simulink model "v3_sim_lqi_sigma_x1_time_variant"  (R2023b)
settings: Solver=VariableStepAuto  StartTime=0.0  StopTime=180  RelTol=1e-10
values from neighbouring files (symbols this model uses):
  K_sigma = [K_sigma, K.']    [WP5.m]
  sigma = [0.01:0.02:2]    [WP5.m]
undefined symbols (not defined in the file or in its folder): reference_selector
libraries: simulink x3
settings Model: Creator=kiraa  LastModifiedBy=kiraa

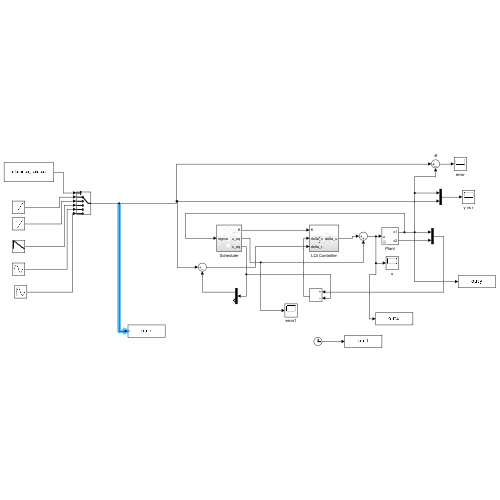
[thumbnail: Simulink's stored preview of the top-level diagram]
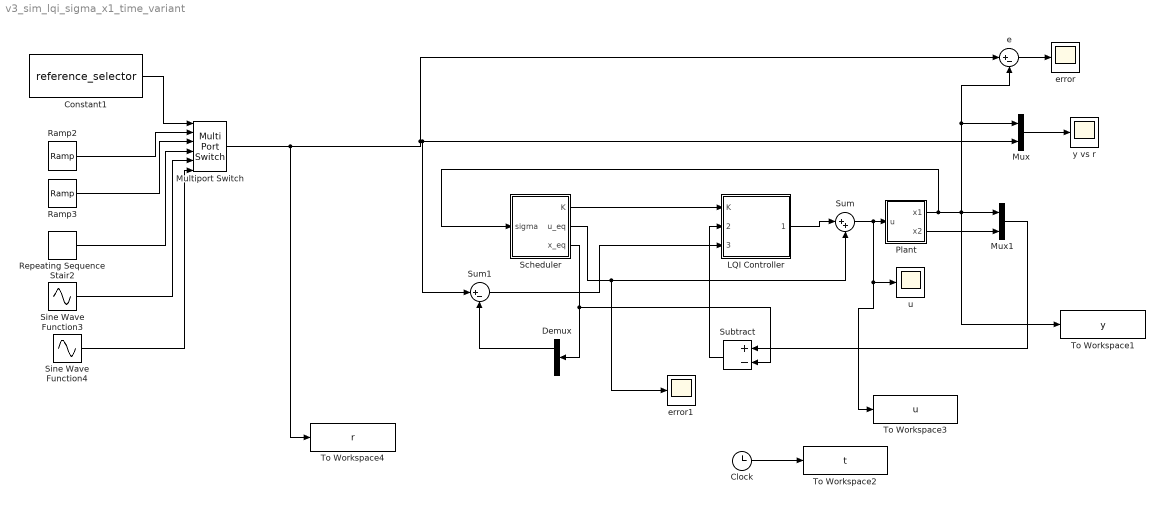
== system v3_sim_lqi_sigma_x1_time_variant ==
  Clock : Clock
  Constant1 : Constant  Value=reference_selector
  Demux : Demux  Outputs=2
  LQI Controller : Subsystem
  Multiport Switch : MultiPortSwitch  Inputs=5  SaturateOnIntegerOverflow=off  InputSameDT=off
  Mux : Mux  Inputs=2
  Mux1 : Mux  Inputs=2
  Plant : Subsystem  mask{x1_0=0.1, x2_0=0}
      mask prompts: x1_0 "x1(0) [g/l]"; x2_0 "x2(0) [min^-1]"
  Ramp2 : simulink/Sources/Ramp  slope=-0.0005  start=0  InitialOutput=0.1
  Ramp3 : simulink/Sources/Ramp  slope=0.005  start=0  InitialOutput=0.1
  Repeating Sequence Stair2 : simulink/Sources/Repeating Sequence Stair  OutValues=[ 0.085 0.08 0.075 0.07 0.065 0.06 0.055 0.05 0.045 0.04 0.035 0.03].'  tsamp=20  OutMin=[]  OutMax=[]  OutDataTypeStr=double  OutputDataTypeScalingMode=double  OutDataType=fixdt(0,8)  ConRadixGroup=Best Precision: Vector-wise  OutScaling=2^-12
  Scheduler : Subsystem
  Sine Wave Function3 : Sin  Amplitude=0.03  Bias=0.05  Frequency=0.05  SampleTime=0
  Sine Wave Function4 : Sin  Amplitude=0.02  Bias=0.05  Frequency=0.1  SampleTime=0
  Subtract : Sum  Inputs=+-
  Sum : Sum  Inputs=|++
  Sum1 : Sum  Inputs=|+-
  To Workspace1 : ToWorkspace  VariableName=y  SampleTime=-1
  To Workspace2 : ToWorkspace  VariableName=t  SampleTime=-1
  To Workspace3 : ToWorkspace  VariableName=u  SampleTime=-1
  To Workspace4 : ToWorkspace  VariableName=r  SampleTime=-1
  e : Sum  Inputs=|+-
  error : Scope
  error1 : Scope
  u : Scope
  y vs r : Scope
  wires:
  Mux/1 -> y vs r/1
  Plant/1(x1) -> Scheduler/1(sigma), To Workspace1/1, Mux/1, e/2, Mux1/1
  LQI Controller/1(delta_u) -> Sum/1
  e/1 -> error/1
  Sum/1 -> To Workspace3/1, u/1, Plant/1(u)
  Subtract/1 -> LQI Controller/2(delta_x)
  Plant/2(x2) -> Mux1/2
  Mux1/1 -> Subtract/1
  Scheduler/2(u_eq) -> error1/1, Sum/2
  Scheduler/3(x_eq) -> Subtract/2, Demux/1
  Scheduler/1(K) -> LQI Controller/1(K)
  Demux/1 -> Sum1/2
  Sum1/1 -> LQI Controller/3(delta_r)
  Clock/1 -> To Workspace2/1
  Sine Wave Function4/1 -> Multiport Switch/6
  Repeating Sequence Stair2/1 -> Multiport Switch/4
  Constant1/1 -> Multiport Switch/1
  Ramp3/1 -> Multiport Switch/3
  Ramp2/1 -> Multiport Switch/2
  Sine Wave Function3/1 -> Multiport Switch/5
  Multiport Switch/1 -> To Workspace4/1, e/1, Mux/2, Sum1/1

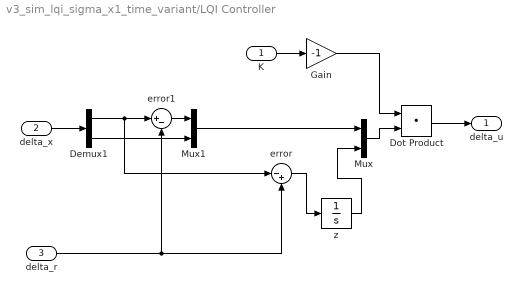
== system v3_sim_lqi_sigma_x1_time_variant/LQI Controller ==
  K : Inport
  delta_x : Inport  Port=2
  delta_r : Inport  Port=3
  Demux1 : Demux  Outputs=2
  Dot Product : DotProduct  OutDataTypeStr=Inherit: Inherit via internal rule
  Gain : Gain  Gain=-1
  Mux : Mux  Inputs=2
  Mux1 : Mux  Inputs=2
  error : Sum  Inputs=|-+
  error1 : Sum  Inputs=|+-
  z : Integrator  InitialCondition=0.1
  delta_u : Outport
  wires:
  Gain/1 -> Dot Product/1
  delta_r/1 -> error1/2, error/2
  Demux1/1 -> error1/1, error/1
  Mux1/1 -> Mux/1
  error/1 -> z/1
  z/1 -> Mux/2
  K/1 -> Gain/1
  Mux/1 -> Dot Product/2
  Dot Product/1 -> delta_u/1
  Demux1/2 -> Mux1/2
  delta_x/1 -> Demux1/1
  error1/1 -> Mux1/1

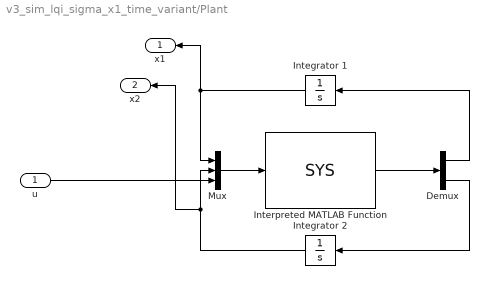
== system v3_sim_lqi_sigma_x1_time_variant/Plant ==
  u : Inport
  Demux : Demux  Outputs=2
  Integrator 1 : Integrator  InitialCondition=x1_0
  Integrator 2 : Integrator  InitialCondition=x2_0
  Interpreted MATLAB Function : MATLABFcn  MATLABFcn=SYS  OutputDimensions=2
  Mux : Mux  Inputs=3
  x1 : Outport
  x2 : Outport  Port=2
  wires:
  Integrator 1/1 -> x1/1, Mux/1
  Demux/1 -> Integrator 1/1
  Mux/1 -> Interpreted MATLAB Function/1
  Integrator 2/1 -> x2/1, Mux/2
  Interpreted MATLAB Function/1 -> Demux/1
  Demux/2 -> Integrator 2/1
  u/1 -> Mux/3

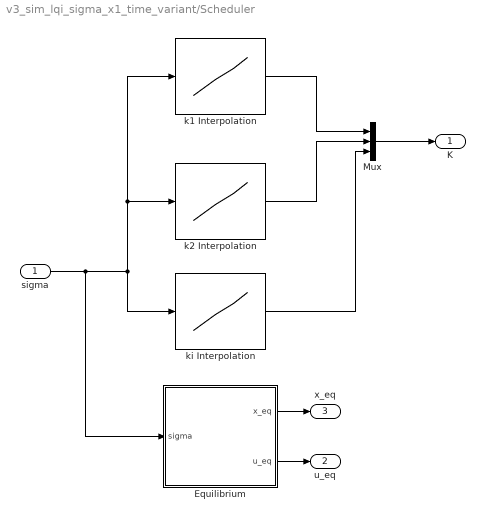
== system v3_sim_lqi_sigma_x1_time_variant/Scheduler ==
  sigma : Inport
  Equilibrium : MATLAB Function  TreatAsAtomicUnit=on
  Mux : Mux  Inputs=3
  k1 Interpolation : Lookup_n-D  NumberOfTableDimensions=1  BreakpointsForDimension1=sigma  Table=K_sigma(1,:)  InternalRulePriority=Speed  OutDataTypeStr=double  RndMeth=Simplest
  k2 Interpolation : Lookup_n-D  NumberOfTableDimensions=1  BreakpointsForDimension1=sigma  Table=K_sigma(2,:)  InternalRulePriority=Speed  OutDataTypeStr=double  RndMeth=Simplest
  ki Interpolation : Lookup_n-D  NumberOfTableDimensions=1  BreakpointsForDimension1=sigma  Table=K_sigma(3,:)  InternalRulePriority=Speed  OutDataTypeStr=double  RndMeth=Simplest
  K : Outport
  u_eq : Outport  Port=2
  x_eq : Outport  Port=3
  wires:
  Equilibrium/1(x_eq) -> x_eq/1
  Equilibrium/2(u_eq) -> u_eq/1
  sigma/1 -> ki Interpolation/1, k1 Interpolation/1, k2 Interpolation/1, Equilibrium/1(sigma)
  k1 Interpolation/1 -> Mux/1
  k2 Interpolation/1 -> Mux/2
  Mux/1 -> K/1
  ki Interpolation/1 -> Mux/3

== matlab function v3_sim_lqi_sigma_x1_time_variant/Scheduler/Equilibrium ==
  data: sigma input; x_eq output; u_eq output
function [x_eq,u_eq] = compute_equilibrium(sigma)
    u_eq = -(399496308545527218176*sigma - 412936040625518808125)/(8736983277098762240000*sigma);
    x_eq = [sigma; -(1360087087465889792*sigma - 1319284474841913125)/(90071992547409920000*sigma)];
end
